simulink model "SineCosine_multiply_input"  (R2021a)
settings: Solver=VariableStepAuto  StartTime=0.0  StopTime=5120  RelTol=1e-3
settings Model: Creator=YOURI  LastModifiedBy=YOURI

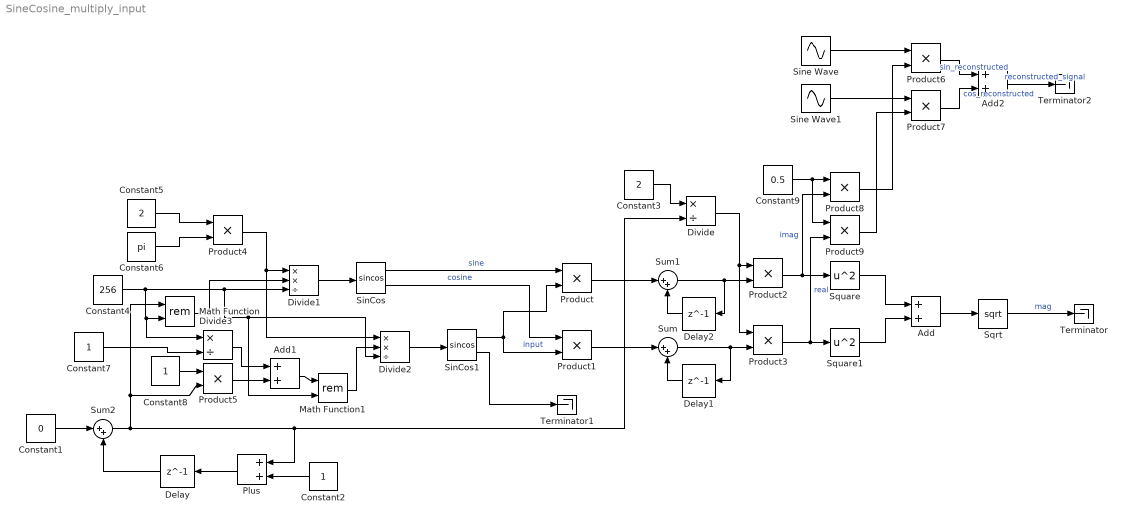
== system SineCosine_multiply_input ==
  Add : Sum
  Add1 : Sum
  Add2 : Sum
  Constant1 : Constant  Value=0
  Constant2 : Constant
  Constant3 : Constant  Value=2
  Constant4 : Constant  Value=256
  Constant5 : Constant  Value=2
  Constant6 : Constant  Value=pi
  Constant7 : Constant
  Constant8 : Constant
  Constant9 : Constant  Value=0.5
  Delay : Delay  DelayLength=1  SampleTime=1
  Delay1 : Delay  DelayLength=1  InitialCondition=0
  Delay2 : Delay  DelayLength=1  InitialCondition=0
  Divide : Product  Inputs=*/
  Divide1 : Product  Inputs=**/
  Divide2 : Product  Inputs=**/
  Divide3 : Product  Inputs=*/
  Math Function : Math  Operator=rem  SaturateOnIntegerOverflow=on
  Math Function1 : Math  Operator=rem  SaturateOnIntegerOverflow=on
  Plus : Sum
  Product{,1..9} (10 alike) : Product
  SinCos : Trigonometry  Operator=sincos  ApproximationMethod=Lookup  NumberOfDataPoints=256
  SinCos1 : Trigonometry  Operator=sincos  ApproximationMethod=Lookup  NumberOfDataPoints=256
  Sine Wave : Sin  Samples=256  SampleTime=0.001
  Sine Wave1 : Sin  Phase=pi/2  Samples=256  SampleTime=0.001  Offset=256/4
  Sqrt : Sqrt  SaturateOnIntegerOverflow=on
  Square : Math  Operator=square  SaturateOnIntegerOverflow=on
  Square1 : Math  Operator=square  SaturateOnIntegerOverflow=on
  Sum : Sum  Inputs=|++
  Sum1 : Sum  Inputs=|++
  Sum2 : Sum  Inputs=|++
  Terminator : Terminator
  Terminator1 : Terminator
  Terminator2 : Terminator
  wires:
  Product1/1 -> Sum/1
  Product/1 -> Sum1/1
  Sum1/1 -> Delay2/1, Product2/2
  Sum/1 -> Delay1/1, Product3/2
  Divide/1 -> Product3/1, Product2/1
  Product3/1 -> Product9/2, Square1/1  "real"
  Product2/1 -> Product8/2, Square/1  "imag"
  Square/1 -> Add/1
  Square1/1 -> Add/2
  Add/1 -> Sqrt/1
  Sqrt/1 -> Terminator/1  "mag"
  Delay1/1 -> Sum/2
  Delay2/1 -> Sum1/2
  Constant1/1 -> Sum2/1
  Plus/1 -> Delay/1
  Sum2/1 -> Product5/2, Math Function/1, Divide/2, Plus/1
  Constant2/1 -> Plus/2
  Constant3/1 -> Divide/1
  Delay/1 -> Sum2/2
  Divide1/1 -> SinCos/1
  Product4/1 -> Divide2/1, Divide1/1
  Constant5/1 -> Product4/1
  Constant6/1 -> Product4/2
  SinCos/1 -> Product/1  "sine"
  SinCos/2 -> Product1/1  "cosine"
  Divide2/1 -> SinCos1/1
  Constant8/1 -> Product5/1
  SinCos1/1 -> Product1/2, Product/2  "input"
  SinCos1/2 -> Terminator1/1
  Constant4/1 -> Divide3/1, Math Function/2, Math Function1/2, Divide2/3, Divide1/3
  Math Function/1 -> Divide1/2
  Math Function1/1 -> Divide2/2
  Add1/1 -> Math Function1/1
  Product5/1 -> Add1/2
  Divide3/1 -> Add1/1
  Constant7/1 -> Divide3/2
  Sine Wave1/1 -> Product7/1
  Sine Wave/1 -> Product6/1
  Product6/1 -> Add2/1  "sin_reconstructed"
  Product7/1 -> Add2/2  "cos_reconstructed"
  Add2/1 -> Terminator2/1  "reconstructed_signal"
  Product8/1 -> Product6/2
  Constant9/1 -> Product9/1, Product8/1
  Product9/1 -> Product7/2
